simulink model "Sim"  (R2021a)
settings: Solver=FixedStepAuto  StartTime=0.0  StopTime=tf  FixedStep=Ts  RelTol=1e-3
values from neighbouring files (symbols this model uses):
  Ts = 0.001    [params.m]
  TWindow = Ts*Nw    (= 0.1)    [params.m]
undefined symbols (not defined in the file or in its folder): Noise
libraries: simulink x1
settings Model: Creator=perruquetti  LastModifiedBy=perruquetti

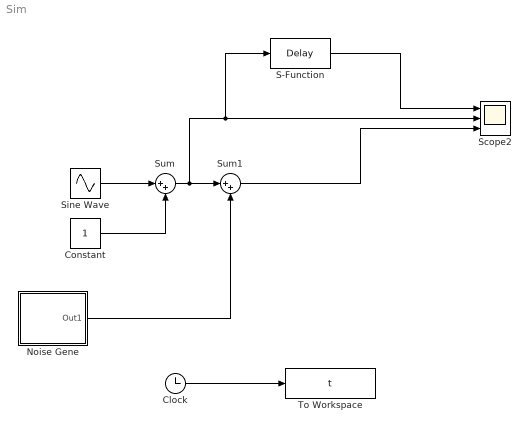
== system Sim ==
  Clock : Clock
  Constant : Constant
  Noise Gene : Subsystem
  S-Function : S-Function  FunctionName=Delay  Parameters=Ts,TWindow  SFunctionDeploymentMode=off  EnableBusSupport=off
  Scope2 : Scope  NumInputPorts=3
  Sine Wave : Sin  Frequency=10  SampleTime=0
  Sum : Sum  Inputs=|++
  Sum1 : Sum  Inputs=|++
  To Workspace : ToWorkspace  VariableName=t  SampleTime=-1
  wires:
  Constant/1 -> Sum/2
  Sine Wave/1 -> Sum/1
  Clock/1 -> To Workspace/1
  Noise Gene/1(Out1) -> Sum1/2
  Sum1/1 -> Scope2/3
  Sum/1 -> S-Function/1, Scope2/2, Sum1/1
  S-Function/1 -> Scope2/1

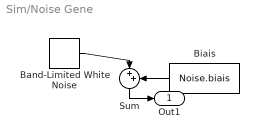
== system Sim/Noise Gene ==
  Band-Limited White Noise : simulink/Sources/Band-Limited White Noise  Cov=Noise.power  Ts=Noise.sampling  seed=Noise.seed
  Biais : Constant  Value=Noise.biais
  Sum : Sum  Inputs=|++
  Out1 : Outport
  wires:
  Sum/1 -> Out1/1
  Biais/1 -> Sum/2
  Band-Limited White Noise/1 -> Sum/1
